simulink model "smartCart5_1work"  (R2016a)
settings: Solver=FixedStepDiscrete  StartTime=0.0  StopTime=inf  FixedStep=1  RelTol=1e-3
libraries: simulink x213, hdlsllib x84
(part 3 of 4)

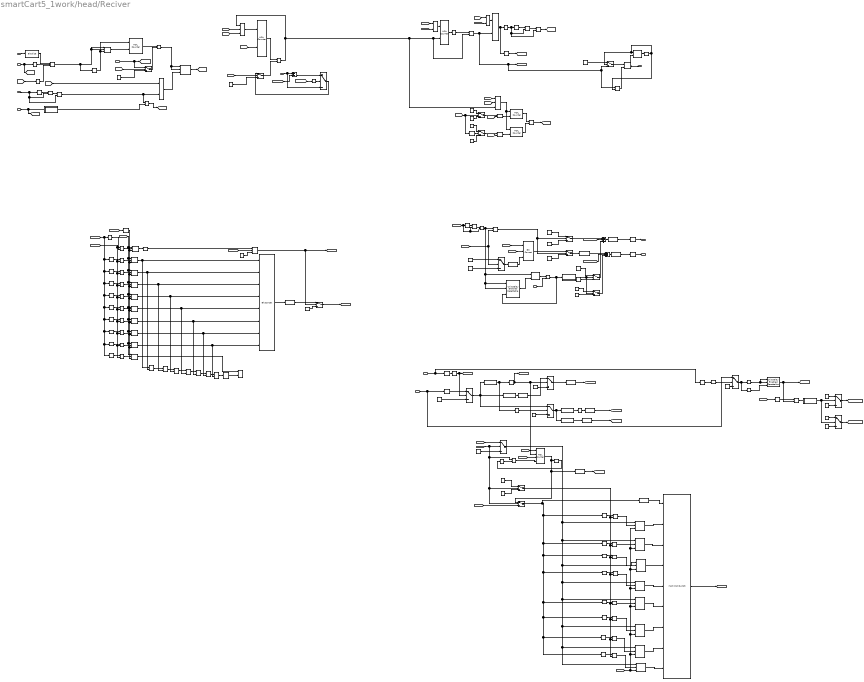
== system smartCart5_1work/head/Reciver ==
  note: Cхема формирования байта и проверка четности
  note: Схема связи (5)
  note: Схема формирования отчёта о работе приёмника (4)
  note: cхема управления и синхронизации (2)
  note: Схема обнаружение сообщения (1)
  RST : Inport  OutDataTypeStr=fixdt(1,3,0)
  IO : Inport  Port=2  OutDataTypeStr=boolean
  STOP : Inport  Port=3  OutDataTypeStr=boolean
  adr_IN : Inport  Port=4  OutDataTypeStr=uint8
  data_in : Inport  Port=5  OutDataTypeStr=uint32
  ON_RECIVER : Inport  Port=6  OutDataTypeStr=boolean
  TimOUT : Inport  Port=7  OutDataTypeStr=uint32
  time_transmite : Inport  Port=8  OutDataTypeStr=uint32
  time_transition : Inport  Port=9  OutDataTypeStr=uint32
  Add : Sum  Inputs=+++
  Add1 : Sum  Inputs=+++
  Add2 : Sum  Inputs=+-
  Bit Concat : hdlsllib/HDL Operations/Bit Concat  numInputs=8
  Bit Concat1 : hdlsllib/HDL Operations/Bit Concat  numInputs=3
  Bit Slice1 : hdlsllib/HDL Operations/Bit Slice  lidx=2  ridx=2
  Bit Slice2 : hdlsllib/HDL Operations/Bit Slice  lidx=1  ridx=0
  Bit Slice3 : hdlsllib/HDL Operations/Bit Slice  lidx=7  ridx=2
  Bit Slice4 : hdlsllib/HDL Operations/Bit Slice  lidx=2  ridx=2
  Bit Slice5 : hdlsllib/HDL Operations/Bit Slice  lidx=8  ridx=3
  Compare To Constant{1,3..4,13,21,31..33} (8 alike) : simulink/Logic and Bit Operations/Compare To Constant  relop===  const=0  OutDataTypeStr=boolean
  Compare To Constant10 : simulink/Logic and Bit Operations/Compare To Constant  relop===  const=7  OutDataTypeStr=boolean
  Compare To Constant11 : simulink/Logic and Bit Operations/Compare To Constant  relop===  const=8  OutDataTypeStr=boolean
  Compare To Constant12 : simulink/Logic and Bit Operations/Compare To Constant  relop===  const=9  OutDataTypeStr=boolean
  Compare To Constant14 : simulink/Logic and Bit Operations/Compare To Constant  relop===  const=6  OutDataTypeStr=boolean
  Compare To Constant15 : simulink/Logic and Bit Operations/Compare To Constant  relop===  const=7  OutDataTypeStr=boolean
  Compare To Constant{5,16,18,20,22,30} (6 alike) : simulink/Logic and Bit Operations/Compare To Constant  relop===  const=1  OutDataTypeStr=boolean
  Compare To Constant17 : simulink/Logic and Bit Operations/Compare To Constant  relop===  const=200  OutDataTypeStr=boolean
  Compare To Constant19 : simulink/Logic and Bit Operations/Compare To Constant  relop===  const=2  OutDataTypeStr=boolean
  Compare To Constant2 : simulink/Logic and Bit Operations/Compare To Constant  relop===  const=10  OutDataTypeStr=boolean
  Compare To Constant23 : simulink/Logic and Bit Operations/Compare To Constant  relop===  const=2  OutDataTypeStr=boolean
  Compare To Constant24 : simulink/Logic and Bit Operations/Compare To Constant  relop===  const=3  OutDataTypeStr=boolean
  Compare To Constant25 : simulink/Logic and Bit Operations/Compare To Constant  relop===  const=4  OutDataTypeStr=boolean
  Compare To Constant26 : simulink/Logic and Bit Operations/Compare To Constant  relop===  const=5  OutDataTypeStr=boolean
  Compare To Constant27 : simulink/Logic and Bit Operations/Compare To Constant  relop===  const=6  OutDataTypeStr=boolean
  Compare To Constant28 : simulink/Logic and Bit Operations/Compare To Constant  relop===  const=7  OutDataTypeStr=boolean
  Compare To Constant29 : simulink/Logic and Bit Operations/Compare To Constant  relop===  const=5  OutDataTypeStr=boolean
  Compare To Constant6 : simulink/Logic and Bit Operations/Compare To Constant  relop===  const=2  OutDataTypeStr=boolean
  Compare To Constant7 : simulink/Logic and Bit Operations/Compare To Constant  relop===  const=3  OutDataTypeStr=boolean
  Compare To Constant8 : simulink/Logic and Bit Operations/Compare To Constant  relop===  const=4  OutDataTypeStr=boolean
  Compare To Constant9 : simulink/Logic and Bit Operations/Compare To Constant  relop===  const=5  OutDataTypeStr=boolean
  Constant{,1,12,20} (4 alike) : Constant  Value=0  OutDataTypeStr=uint8
  Constant10 : Constant  Value=0  OutDataTypeStr=boolean  SampleTime=-1
  Constant11 : Constant  Value=0  OutDataTypeStr=boolean
  Constant{3,7,13..15} (5 alike) : Constant  Value=0  OutDataTypeStr=uint32  SampleTime=-1
  Constant16 : Constant  Value=0  OutDataTypeStr=uint8  SampleTime=-1
  Constant17 : Constant  Value=5  OutDataTypeStr=uint8  SampleTime=-1
  Constant18 : Constant  OutDataTypeStr=uint8  SampleTime=-1
  Constant19 : Constant  Value=6  OutDataTypeStr=uint8
  Constant2 : Constant  OutDataTypeStr=uint8
  Constant21 : Constant  Value=0  OutDataTypeStr=uint32
  Constant22 : Constant  OutDataTypeStr=uint32
  Constant23 : Constant  OutDataTypeStr=uint32  SampleTime=-1
  Constant24 : Constant  OutDataTypeStr=uint32  SampleTime=-1
  Constant26 : Constant  OutDataTypeStr=boolean  SampleTime=-1
  Constant27 : Constant  OutDataTypeStr=boolean  SampleTime=-1
  Constant28 : Constant  Value=0  OutDataTypeStr=boolean  SampleTime=-1
  Constant29 : Constant  Value=0  OutDataTypeStr=boolean  SampleTime=-1
  Constant4 : Constant  Value=2  OutDataTypeStr=fixdt(0,2,0)
  Constant5 : Constant  Value=0  OutDataTypeStr=uint8  SampleTime=-1
  Constant6 : Constant  OutDataTypeStr=boolean
  Constant8 : Constant  OutDataTypeStr=fixdt(0,2,0)
  Constant9 : Constant  OutDataTypeStr=boolean
  Data Type Conversion : DataTypeConversion  OutDataTypeStr=uint8
  Data Type Conversion1 : DataTypeConversion  OutDataTypeStr=fixdt(0,5,0)
  Data Type Conversion10 : DataTypeConversion  OutDataTypeStr=uint8
  Data Type Conversion2 : DataTypeConversion  OutDataTypeStr=uint8
  Data Type Conversion3 : DataTypeConversion  OutDataTypeStr=boolean
  Data Type Conversion4 : DataTypeConversion  OutDataTypeStr=uint32
  Data Type Conversion5 : DataTypeConversion  OutDataTypeStr=uint32
  Data Type Conversion6 : DataTypeConversion  OutDataTypeStr=fixdt(0,5,0)
  Data Type Conversion7 : DataTypeConversion  OutDataTypeStr=fixdt(0,2,0)
  Data Type Conversion8 : DataTypeConversion  OutDataTypeStr=fixdt(1,4,0)
  Data Type Conversion9 : DataTypeConversion  OutDataTypeStr=uint32
  Delay{1..9,11} (10 alike) : Delay  DelayLength=1  InitialCondition=0
  HDL Counter{,6,8..9} (4 alike) : hdlsllib/HDL Operations/HDL Counter  CountType=Free running  CountInit=0  CountStep=1  CountMax=1  CountFromType=Initial value  CountFrom=0  CountResetPort=on  CountLoadPort=off  CountEnbPort=on  CountDirPort=off  CountDataType=Unsigned  CountWordLen=32  CountFracLen=0  CountSampTime=1
  HDL Counter1 : hdlsllib/HDL Operations/HDL Counter  CountType=Free running  CountInit=0  CountStep=1  CountMax=1  CountFromType=Initial value  CountFrom=0  CountResetPort=on  CountLoadPort=off  CountEnbPort=on  CountDirPort=off  CountDataType=Unsigned  CountWordLen=1  CountFracLen=0  CountSampTime=1
  HDL Counter2 : hdlsllib/HDL Operations/HDL Counter  CountType=Count limited  CountInit=0  CountStep=1  CountMax=10  CountFromType=Initial value  CountFrom=0  CountResetPort=on  CountLoadPort=off  CountEnbPort=on  CountDirPort=off  CountDataType=Unsigned  CountWordLen=4  CountFracLen=0  CountSampTime=1
  HDL Counter3 : hdlsllib/HDL Operations/HDL Counter  CountType=Free running  CountInit=0  CountStep=1  CountMax=1  CountFromType=Initial value  CountFrom=0  CountResetPort=on  CountLoadPort=on  CountEnbPort=on  CountDirPort=off  CountDataType=Unsigned  CountWordLen=5  CountFracLen=0  CountSampTime=1
  HDL Counter4 : hdlsllib/HDL Operations/HDL Counter  CountType=Free running  CountInit=0  CountStep=1  CountMax=1  CountFromType=Initial value  CountFrom=0  CountResetPort=on  CountLoadPort=off  CountEnbPort=on  CountDirPort=off  CountDataType=Unsigned  CountWordLen=8  CountFracLen=0  CountSampTime=1
  HDL Counter5 : hdlsllib/HDL Operations/HDL Counter  CountType=Free running  CountInit=0  CountStep=1  CountMax=25  CountFromType=Initial value  CountFrom=0  CountResetPort=on  CountLoadPort=off  CountEnbPort=on  CountDirPort=off  CountDataType=Unsigned  CountWordLen=32  CountFracLen=0  CountSampTime=1
  Index Vector : MultiPortSwitch  DataPortOrder=Zero-based contiguous  Inputs=8  zeroidx=on
  Logical Operator{,7,9,12..21,33,36,38..46,49..50} (26 alike) : Logic  AllPortsSameDT=off  OutDataTypeStr=boolean
  Logical Operator{1,10..11,34..35,48} (6 alike) : Logic  Operator=OR  AllPortsSameDT=off  OutDataTypeStr=boolean
  Logical Operator2 : Logic  Operator=NOT  Inputs=3  AllPortsSameDT=off  OutDataTypeStr=boolean
  Logical Operator22 : Logic  Inputs=3  AllPortsSameDT=off  OutDataTypeStr=boolean
  Logical Operator{5..6,23..24,26..30,32} (10 alike) : Logic  Operator=XOR  AllPortsSameDT=off  OutDataTypeStr=boolean
  Logical Operator25 : Logic  Inputs=3  AllPortsSameDT=off  OutDataTypeStr=boolean
  Logical Operator31 : Logic  Operator=NOT  AllPortsSameDT=off  OutDataTypeStr=boolean
  Logical Operator37 : Logic  Operator=NOT  AllPortsSameDT=off  OutDataTypeStr=boolean
  Logical Operator4 : Logic  Operator=NOT  Inputs=3  AllPortsSameDT=off  OutDataTypeStr=boolean
  Logical Operator47 : Logic  Operator=NOT  Inputs=3  AllPortsSameDT=off  OutDataTypeStr=boolean
  Logical Operator51 : Logic  Operator=OR  Inputs=3  AllPortsSameDT=off  OutDataTypeStr=boolean
  Logical Operator8 : Logic  Operator=OR  Inputs=3  AllPortsSameDT=off  OutDataTypeStr=boolean
  Relational Operator{,1..3} (4 alike) : RelationalOperator  Operator===  OutDataTypeStr=boolean
  Relational Operator5 : RelationalOperator  Operator=>  OutDataTypeStr=boolean
  SA12 : simulink/Additional Math & Discrete/Additional Discrete/Unit Delay Enabled  vinit=0  tsamp=-1
  Switch{,1..18,20..21} (21 alike) : Switch  Criteria=u2 ~= 0
  Unit Delay Enabled Resettable{,1..21} (22 alike) : simulink/Additional Math & Discrete/Additional Discrete/Unit Delay Enabled Resettable  vinit=0.0  tsamp=-1
  signal_edg : Subsystem  TreatAsAtomicUnit=on
  signal_edg5 : Subsystem  TreatAsAtomicUnit=on
  signal_edg6 : Subsystem  TreatAsAtomicUnit=on
  AddrOUT : Outport  OutDataTypeStr=uint8
  STATUS : Outport  Port=2  OutDataTypeStr=uint32
  Strob : Outport  Port=3  OutDataTypeStr=boolean
  wires:
  RST/1 -> Bit Slice1/1
  Bit Slice1/1 -> Logical Operator25/1
  [bait_done] -> Logical Operator1/1
  Logical Operator1/1 -> Unit Delay Enabled Resettable/3
  Unit Delay Enabled Resettable/1 -> [Mes_res]
  HDL Counter/1 -> Relational Operator2/1
  Relational Operator2/1 -> Logical Operator8/1, Logical Operator51/3, HDL Counter1/2, Logical Operator/2
  HDL Counter1/1 -> Compare To Constant1/1
  Compare To Constant1/1 -> Logical Operator/1
  HDL Counter2/1 -> Delay3/1, Compare To Constant2/1
  Compare To Constant2/1 -> Logical Operator7/2, Logical Operator6/2, Delay2/1
  Delay2/1 -> Logical Operator6/1
  Logical Operator6/1 -> Logical Operator7/1
  Logical Operator8/1 -> HDL Counter/1
  Logical Operator7/1 -> [bait_done]
  [bait_done] -> Logical Operator8/2
  [Mes_res] -> HDL Counter/2
  Delay1/1 -> Logical Operator5/1
  Logical Operator5/1 -> Logical Operator9/1
  STOP/1 -> Logical Operator9/2, Logical Operator5/2, Delay1/1
  Logical Operator9/1 -> Logical Operator48/1, Logical Operator1/2
  [RST] -> Logical Operator8/3
  Logical Operator10/1 -> HDL Counter1/1
  [bait_done] -> Logical Operator10/1
  [RST] -> Logical Operator10/2
  Logical Operator11/1 -> HDL Counter2/1
  [bait_done] -> Logical Operator11/1
  [RST] -> Logical Operator11/2
  Delay3/1 -> [Number_bit]
  Compare To Constant5/1 -> Logical Operator13/1
  Compare To Constant6/1 -> Logical Operator14/1
  Logical Operator14/1 -> Unit Delay Enabled Resettable3/2
  Compare To Constant7/1 -> Logical Operator15/1
  Compare To Constant8/1 -> Logical Operator16/1
  Compare To Constant9/1 -> Logical Operator17/1
  Logical Operator17/1 -> Unit Delay Enabled Resettable6/2
  Compare To Constant14/1 -> Logical Operator18/1
  Logical Operator18/1 -> Unit Delay Enabled Resettable7/2
  Compare To Constant10/1 -> Logical Operator19/1
  Compare To Constant11/1 -> Logical Operator20/1
  Compare To Constant12/1 -> Logical Operator21/1
  [Number_bit] -> Compare To Constant12/1, Compare To Constant11/1, Compare To Constant10/1, Compare To Constant14/1, Compare To Constant9/1, Compare To Constant8/1, Compare To Constant7/1, Compare To Constant6/1, Compare To Constant5/1, Compare To Constant3/1
  Unit Delay Enabled Resettable1/1 -> Compare To Constant13/1
  Compare To Constant13/1 -> Logical Operator22/1
  Compare To Constant3/1 -> Logical Operator12/2
  [Get_val] -> Logical Operator17/2, Logical Operator21/2, Logical Operator20/2, Logical Operator19/2, Logical Operator18/2, Logical Operator16/2, Logical Operator15/2, Logical Operator14/2, Logical Operator13/2, Logical Operator12/1
  [bait_done] -> Logical Operator22/2
  Unit Delay Enabled Resettable3/1 -> Logical Operator23/2, Bit Concat/2
  Unit Delay Enabled Resettable4/1 -> Logical Operator24/2, Bit Concat/3
  Unit Delay Enabled Resettable5/1 -> Logical Operator26/2, Bit Concat/4
  Unit Delay Enabled Resettable6/1 -> Logical Operator27/2, Bit Concat/5
  Unit Delay Enabled Resettable7/1 -> Logical Operator28/2, Bit Concat/6
  Unit Delay Enabled Resettable8/1 -> Logical Operator29/2, Bit Concat/7
  Unit Delay Enabled Resettable9/1 -> Logical Operator30/2, Bit Concat/8
  Unit Delay Enabled Resettable2/1 -> Logical Operator23/1, Bit Concat/1
  Logical Operator23/1 -> Logical Operator24/1
  Logical Operator24/1 -> Logical Operator26/1
  Logical Operator26/1 -> Logical Operator27/1
  Logical Operator27/1 -> Logical Operator28/1
  Logical Operator28/1 -> Logical Operator29/1
  Logical Operator29/1 -> Logical Operator30/1
  Logical Operator30/1 -> Logical Operator31/1
  Bit Concat/1 -> Data Type Conversion/1
  Logical Operator31/1 -> Relational Operator/2
  Unit Delay Enabled Resettable10/1 -> Relational Operator/1
  Logical Operator22/1 -> Switch1/2, [Error_bait]
  Data Type Conversion/1 -> Switch1/1
  Constant/1 -> Switch1/3
  Constant1/1 -> Switch2/3
  Constant2/1 -> Switch2/1
  Constant5/1 -> Switch4/3
  [Error_bait] -> Logical Operator36/1, Switch6/2, Switch5/2, Switch4/2
  [bait] -> Switch4/1
  HDL Counter3/1 -> Switch6/1, Data Type Conversion2/1, Compare To Constant15/1
  Logical Operator36/1 -> HDL Counter3/4
  Compare To Constant15/1 -> Logical Operator37/1
  Logical Operator37/1 -> Logical Operator36/2
  Data Type Conversion2/1 -> [Num_Count]
  Logical Operator35/1 -> Switch2/2, Switch3/2
  Delay5/1 -> Unit Delay Enabled Resettable10/3, Unit Delay Enabled Resettable9/3, Unit Delay Enabled Resettable8/3, Unit Delay Enabled Resettable7/3, Unit Delay Enabled Resettable6/3, Unit Delay Enabled Resettable5/3, Unit Delay Enabled Resettable4/3, Unit Delay Enabled Resettable3/3, Unit Delay Enabled Resettable2/3, Unit Delay Enabled Resettable1/3
  [bait_done] -> Delay5/1
  Logical Operator13/1 -> Unit Delay Enabled Resettable2/2
  Logical Operator12/1 -> Unit Delay Enabled Resettable1/2
  Logical Operator15/1 -> Unit Delay Enabled Resettable4/2
  Logical Operator16/1 -> Unit Delay Enabled Resettable5/2
  Logical Operator19/1 -> Unit Delay Enabled Resettable8/2
  Logical Operator21/1 -> Unit Delay Enabled Resettable10/2
  [data] -> Unit Delay Enabled Resettable10/1, Unit Delay Enabled Resettable9/1, Unit Delay Enabled Resettable8/1, Unit Delay Enabled Resettable7/1, Unit Delay Enabled Resettable6/1, Unit Delay Enabled Resettable5/1, Unit Delay Enabled Resettable4/1, Unit Delay Enabled Resettable3/1, Unit Delay Enabled Resettable2/1, Unit Delay Enabled Resettable1/1
  Logical Operator20/1 -> Unit Delay Enabled Resettable9/2
  Logical Operator/1 -> Logical Operator34/1, Switch8/3, [Get_val], HDL Counter2/2
  Switch8/1 -> SA12/1
  Constant10/1 -> Switch8/1
  SA12/1 -> Strob/1, HDL Counter4/2
  HDL Counter4/1 -> Compare To Constant17/1
  Compare To Constant17/1 -> Switch8/2, HDL Counter4/1, Logical Operator34/2
  Logical Operator34/1 -> SA12/2
  Constant11/1 -> Switch5/3
  Constant6/1 -> Switch5/1
  [addRd] -> Switch6/3
  Constant9/1 -> Logical Operator22/3
  Index Vector/1 -> [Read_Byte]
  Bit Concat1/1 -> Switch3/1
  Switch3/1 -> Data Type Conversion4/1
  [Num_Count] -> Bit Concat1/2
  Constant12/1 -> Switch3/3
  Bit Slice2/1 -> Compare To Constant19/1, Compare To Constant18/1
  Bit Slice3/1 -> Data Type Conversion5/1
  Data Type Conversion5/1 -> Switch7/1
  Constant3/1 -> Switch7/3
  Switch7/1 -> Data Type Conversion6/1
  Data Type Conversion6/1 -> [VAL_COUNT]
  Compare To Constant16/1 -> Switch11/2, [Send_com]
  Compare To Constant18/1 -> [WE], Switch7/2, HDL Counter3/2
  [VAL_COUNT] -> HDL Counter3/3
  Compare To Constant19/1 -> Switch9/2
  Constant7/1 -> Switch9/3
  Switch9/1 -> Bit Slice5/1, Bit Slice4/1
  Bit Slice4/1 -> Compare To Constant20/1
  Compare To Constant20/1 -> Data Type Conversion3/1
  Data Type Conversion3/1 -> [RD]
  Bit Slice5/1 -> Data Type Conversion1/1
  Data Type Conversion1/1 -> [addRd]
  Constant4/1 -> Switch10/1
  Constant8/1 -> Switch10/3
  Switch10/1 -> Data Type Conversion7/1
  Data Type Conversion7/1 -> Bit Concat1/3
  Delay7/1 -> Compare To Constant16/1
  adr_IN/1 -> Delay9/1, Delay7/1
  data_in/1 -> Switch12/1, Delay11/1
  Switch11/1 -> Bit Slice2/1, Switch9/1, Bit Slice3/1
  [Error_bait] -> Logical Operator32/2, Logical Operator33/2, Delay4/1
  Delay4/1 -> Logical Operator32/1
  Logical Operator32/1 -> Logical Operator33/1
  Logical Operator33/1 -> Unit Delay Enabled Resettable20/1, Unit Delay Enabled Resettable20/2, HDL Counter5/1, Logical Operator35/1
  Delay11/1 -> Switch11/1
  Constant14/1 -> Switch11/3
  [Read_Byte] -> Bit Concat1/1
  [RD] -> Switch10/2, Logical Operator35/2
  Compare To Constant21/1 -> Logical Operator39/1
  Logical Operator39/1 -> Unit Delay Enabled Resettable11/2
  Compare To Constant22/1 -> Logical Operator40/1
  Logical Operator40/1 -> Unit Delay Enabled Resettable12/2
  Compare To Constant23/1 -> Logical Operator41/1
  Logical Operator41/1 -> Unit Delay Enabled Resettable13/2
  Compare To Constant24/1 -> Logical Operator42/1
  Logical Operator42/1 -> Unit Delay Enabled Resettable14/2
  Compare To Constant25/1 -> Logical Operator43/1
  Logical Operator43/1 -> Unit Delay Enabled Resettable15/2
  Compare To Constant26/1 -> Logical Operator44/1
  Logical Operator44/1 -> Unit Delay Enabled Resettable16/2
  Compare To Constant27/1 -> Logical Operator45/1
  Logical Operator45/1 -> Unit Delay Enabled Resettable18/2
  Switch4/1 -> Unit Delay Enabled Resettable19/1, Unit Delay Enabled Resettable18/1, Unit Delay Enabled Resettable16/1, Unit Delay Enabled Resettable15/1, Unit Delay Enabled Resettable14/1, Unit Delay Enabled Resettable13/1, Unit Delay Enabled Resettable12/1, Unit Delay Enabled Resettable11/1
  Compare To Constant28/1 -> Logical Operator46/1
  Logical Operator46/1 -> Unit Delay Enabled Resettable19/2
  Unit Delay Enabled Resettable19/1 -> Index Vector/9
  Unit Delay Enabled Resettable18/1 -> Index Vector/8
  Unit Delay Enabled Resettable16/1 -> Index Vector/7
  Unit Delay Enabled Resettable15/1 -> Index Vector/6
  Unit Delay Enabled Resettable14/1 -> Index Vector/5
  Unit Delay Enabled Resettable13/1 -> Index Vector/4
  Unit Delay Enabled Resettable12/1 -> Index Vector/3
  Unit Delay Enabled Resettable11/1 -> Index Vector/2
  Data Type Conversion8/1 -> Index Vector/1
  Switch6/1 -> Data Type Conversion8/1, Compare To Constant28/1, Compare To Constant27/1, Compare To Constant26/1, Compare To Constant25/1, Compare To Constant24/1, Compare To Constant23/1, Compare To Constant22/1, Compare To Constant21/1
  Switch5/1 -> Logical Operator46/2, Logical Operator45/2, Logical Operator44/2, Logical Operator43/2, Logical Operator42/2, Logical Operator41/2, Logical Operator40/2, Logical Operator39/2
  [RST] -> Unit Delay Enabled Resettable13/3, Unit Delay Enabled Resettable11/3, Unit Delay Enabled Resettable12/3, Unit Delay Enabled Resettable14/3, Unit Delay Enabled Resettable15/3, Unit Delay Enabled Resettable16/3, Unit Delay Enabled Resettable18/3, Unit Delay Enabled Resettable19/3
  Delay9/1 -> Compare To Constant29/1
  Compare To Constant29/1 -> Switch12/2
  Constant13/1 -> Switch12/3
  Switch12/1 -> Compare To Constant32/1, Compare To Constant30/1
  Compare To Constant30/1 -> Unit Delay Enabled Resettable17/1, Unit Delay Enabled Resettable17/2
  signal_edg/1(Out1) -> Switch14/2, Switch13/2
  Constant15/1 -> Switch14/3
  Constant16/1 -> Switch13/3
  Constant17/1 -> Switch13/1
  Constant18/1 -> Switch14/1
  Compare To Constant32/1 -> Unit Delay Enabled Resettable17/3
  Unit Delay Enabled Resettable17/1 -> Logical Operator38/2, [detect_error]
  [data] -> Compare To Constant31/1
  Compare To Constant31/1 -> Logical Operator38/1
  Logical Operator38/1 -> signal_edg/1(In1)
  [detect_error] -> Logical Operator47/1
  Logical Operator47/1 -> Logical Operator25/3
  Switch13/1 -> [addr_detect_error]
  Switch14/1 -> [data_detect_error]
  Data Type Conversion4/1 -> Add/1
  Switch2/1 -> Add1/1
  [addr_detect_error] -> Add1/2
  [data_detect_error] -> Add/2
  Add/1 -> Data Type Conversion9/1
  Add1/1 -> Data Type Conversion10/1
  Switch1/1 -> [bait]
  ON_RECIVER/1 -> [on_reciver], signal_edg5/1(In1)
  signal_edg5/1(Out1) -> Logical Operator48/2
  Logical Operator48/1 -> [RST]
  [RST] -> HDL Counter3/1
  Unit Delay Enabled Resettable20/1 -> HDL Counter5/2
  HDL Counter5/1 -> Relational Operator1/1
  Relational Operator1/1 -> Unit Delay Enabled Resettable20/3, signal_edg6/1(In1)
  signal_edg6/1(Out1) -> Switch16/2, Switch15/2
  Constant19/1 -> Switch15/1
  Constant20/1 -> Switch15/3
  Constant21/1 -> Switch16/3
  Constant22/1 -> Switch16/1
  Data Type Conversion9/1 -> Delay6/1
  Data Type Conversion10/1 -> Delay8/1
  Delay8/1 -> AddrOUT/1
  Delay6/1 -> STATUS/1
  Switch15/1 -> Add1/3
  Switch16/1 -> Add/3
  TimOUT/1 -> Relational Operator1/2
  Constant23/1 -> Switch/3
  [on_reciver] -> Switch/2
  Switch/1 -> Relational Operator2/2
  Unit Delay Enabled Resettable21/1 -> HDL Counter6/2
  HDL Counter6/1 -> Relational Operator3/1
  Constant24/1 -> Switch17/3
  [on_reciver] -> Switch17/2
  time_transition/1 -> Switch17/1, [time_transition]
  Switch17/1 -> Relational Operator3/2
  Relational Operator3/1 -> Unit Delay Enabled Resettable/1, Unit Delay Enabled Resettable/2
  IO/1 -> [IO], Compare To Constant33/1
  Add2/1 -> Switch18/1
  [time_transition] -> Add2/2
  Compare To Constant4/1 -> Switch18/2
  [Number_bit] -> Compare To Constant4/1
  Logical Operator25/1 -> Logical Operator2/1, Unit Delay Enabled Resettable21/2, Unit Delay Enabled Resettable21/1
  Logical Operator2/1 -> Unit Delay Enabled Resettable21/3, HDL Counter6/1
  Compare To Constant33/1 -> Logical Operator25/2
  time_transmite/1 -> Switch18/3, Add2/1
  Switch18/1 -> Switch/1
  [IO] -> Logical Operator4/1, Switch20/2
  Logical Operator4/1 -> Switch21/2
  Constant26/1 -> Switch20/1
  Constant27/1 -> Switch21/1
  Constant28/1 -> Switch20/3
  Constant29/1 -> Switch21/3
  Switch20/1 -> Logical Operator49/1
  Logical Operator49/1 -> HDL Counter8/2
  [Mes_res] -> Logical Operator49/2
  Switch21/1 -> Logical Operator50/1
  Logical Operator50/1 -> HDL Counter9/2
  [Mes_res] -> Logical Operator50/2
  [RST] -> Logical Operator51/2
  [bait_done] -> Logical Operator51/1
  Logical Operator51/1 -> HDL Counter9/1, HDL Counter8/1
  HDL Counter8/1 -> Relational Operator5/1
  HDL Counter9/1 -> Relational Operator5/2
  Relational Operator5/1 -> [data]

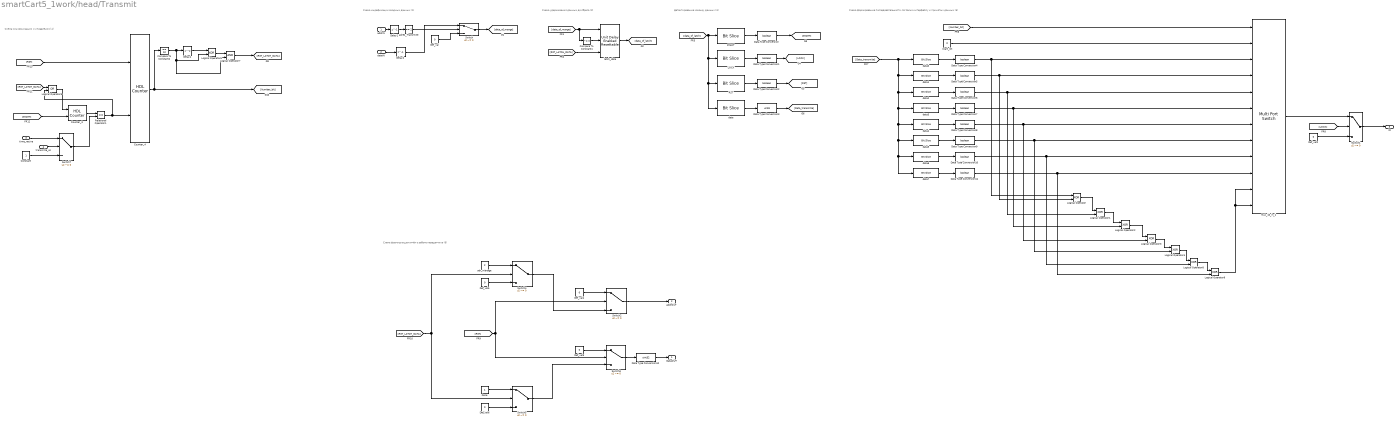
== system smartCart5_1work/head/Transmit ==
  note: Схема формирующая отчёт о работе передатчика (6)
  note: Схема формирование последовательности согласно интерфейсу и принятых данных (5)
  note: Детектирование команд, данных (3)
  note: Схема удерживания данных до сброса (2)
  note: Схема индефикации входных данных (1)
  note: Схема синхронизации и управления (4)
  addrIN : Inport  OutDataTypeStr=uint8
  dataIN : Inport  Port=2  OutDataTypeStr=fixdt(0,32,0)
  time_recive : Inport  Port=3  OutDataTypeStr=uint32
  transmite_on : Inport  Port=4  OutDataTypeStr=boolean
  Compare To Constant1 : simulink/Logic and Bit Operations/Compare To Constant  relop=~=  const=0  OutDataTypeStr=boolean
  Compare To Constant2 : simulink/Logic and Bit Operations/Compare To Constant  relop===  const=10  OutDataTypeStr=boolean
  Constant : Constant  OutDataTypeStr=uint32  SampleTime=-1
  Counter_3 : hdlsllib/HDL Operations/HDL Counter  CountType=Free running  CountInit=0  CountStep=1  CountMax=5208  CountFromType=Initial value  CountFrom=0  CountResetPort=on  CountLoadPort=off  CountEnbPort=on  CountDirPort=off  CountDataType=Unsigned  CountWordLen=32  CountFracLen=0  CountSampTime=1
  Counter_4 : hdlsllib/HDL Operations/HDL Counter  CountType=Count limited  CountInit=0  CountStep=1  CountMax=11  CountFromType=Initial value  CountFrom=0  CountResetPort=on  CountLoadPort=off  CountEnbPort=on  CountDirPort=off  CountDataType=Unsigned  CountWordLen=4  CountFracLen=0  CountSampTime=1
  Data Type Conversion{,1..2,4..11} (11 alike) : DataTypeConversion  OutDataTypeStr=boolean
  Data Type Conversion12 : DataTypeConversion  OutDataTypeStr=uint32
  Data Type Conversion3 : DataTypeConversion  OutDataTypeStr=uint8
  Def_val : Constant  Value=0  OutDataTypeStr=fixdt(0,32,0)  SampleTime=-1
  Def_val2 : Constant  Value=0  OutDataTypeStr=boolean  SampleTime=-1
  Def_val{3..6} (4 alike) : Constant  Value=0  OutDataTypeStr=uint8  SampleTime=-1
  Delay1 : Delay  DelayLength=1  InitialCondition=0
  Delay2 : Delay  DelayLength=1  InitialCondition=0
  Delay4 : Delay
  Done : Constant  OutDataTypeStr=uint8  SampleTime=-1
  LOCK : hdlsllib/HDL Operations/Bit Slice  lidx=1  ridx=1
  Logical Operator{,1..4,6,8..9} (8 alike) : Logic  Operator=XOR  AllPortsSameDT=off  OutDataTypeStr=boolean
  Logical Operator5 : Logic  Operator=OR  AllPortsSameDT=off  OutDataTypeStr=boolean
  Logical Operator7 : Logic  AllPortsSameDT=off  OutDataTypeStr=boolean
  RST : hdlsllib/HDL Operations/Bit Slice  lidx=2  ridx=2
  Relational Operator1 : RelationalOperator  Operator===  OutDataTypeStr=boolean
  START : hdlsllib/HDL Operations/Bit Slice  lidx=0  ridx=0
  Switch{,1..5,7} (7 alike) : Switch  Criteria=u2 ~= 0
  adr_manage : Constant  Value=2  OutDataTypeStr=uint8  SampleTime=-1
  adres_Transmite : simulink/Logic and Bit Operations/Compare To Constant  relop===  const=2  OutDataTypeStr=boolean
  data : hdlsllib/HDL Operations/Bit Slice  lidx=10  ridx=3
  "data0 " : hdlsllib/HDL Operations/Bit Slice  lidx=0  ridx=0
  data1 : hdlsllib/HDL Operations/Bit Slice  lidx=1  ridx=1
  data2 : hdlsllib/HDL Operations/Bit Slice  lidx=2  ridx=2
  data3 : hdlsllib/HDL Operations/Bit Slice  lidx=3  ridx=3
  data4 : hdlsllib/HDL Operations/Bit Slice  lidx=4  ridx=4
  data5 : hdlsllib/HDL Operations/Bit Slice  lidx=5  ridx=5
  data6 : hdlsllib/HDL Operations/Bit Slice  lidx=6  ridx=6
  data7 : hdlsllib/HDL Operations/Bit Slice  lidx=7  ridx=7
  latch_data : simulink/Additional Math & Discrete/Additional Discrete/Unit Delay Enabled Resettable  vinit=0  tsamp=-1
  mux_10_in_1 : MultiPortSwitch  DataPortOrder=Zero-based contiguous  Inputs=11  zeroidx=on
  start_bit : Constant  Value=0  OutDataTypeStr=boolean  SampleTime=-1
  DataOUT : Outport  OutDataTypeStr=uint32
  addrOUT : Outport  Port=2  OutDataTypeStr=uint8
  IO : Outport  Port=3  OutDataTypeStr=boolean
  wires:
  adres_Transmite/1 -> Switch/2
  Def_val/1 -> Switch/3
  START/1 -> Data Type Conversion/1
  LOCK/1 -> Data Type Conversion1/1
  RST/1 -> Data Type Conversion2/1
  data/1 -> Data Type Conversion3/1
  [RST_LATCH_DATA] -> latch_data/3
  Switch/1 -> [data_of_mange]
  latch_data/1 -> [data_of_latch]
  [data_of_latch] -> data/1, RST/1, LOCK/1, START/1
  Data Type Conversion/1 -> [START]
  Data Type Conversion1/1 -> [LOCK]
  Data Type Conversion2/1 -> [RST]
  Compare To Constant1/1 -> latch_data/2
  [Number_bit] -> mux_10_in_1/1
  start_bit/1 -> mux_10_in_1/2
  "data0 "/1 -> Data Type Conversion4/1
  data1/1 -> Data Type Conversion5/1
  data2/1 -> Data Type Conversion6/1
  data3/1 -> Data Type Conversion7/1
  data4/1 -> Data Type Conversion8/1
  data5/1 -> Data Type Conversion9/1
  data6/1 -> Data Type Conversion10/1
  [Data_transmite] -> data7/1, data6/1, data5/1, data4/1, data3/1, data2/1, data1/1, "data0 "/1
  data7/1 -> Data Type Conversion11/1
  mux_10_in_1/1 -> Switch1/1
  [LOCK] -> Switch1/2
  Switch1/1 -> IO/1
  Switch2/1 -> addrOUT/1
  Def_val4/1 -> Switch2/1
  Def_val3/1 -> Switch3/1
  [RST] -> Switch2/2, Switch3/2
  Switch4/1 -> Switch2/3
  Switch5/1 -> Switch3/3
  [RST_LATCH_DATA] -> Switch4/2, Switch5/2
  Def_val5/1 -> Switch4/3
  Def_val6/1 -> Switch5/3
  adr_manage/1 -> Switch4/1
  Done/1 -> Switch5/1
  [data_of_mange] -> latch_data/1, Compare To Constant1/1
  Data Type Conversion3/1 -> [Data_transmite]
  Def_val2/1 -> Switch1/3
  addrIN/1 -> Delay1/1
  Delay1/1 -> adres_Transmite/1
  dataIN/1 -> Delay2/1
  Delay2/1 -> Switch/1
  Data Type Conversion12/1 -> DataOUT/1
  Switch3/1 -> Data Type Conversion12/1
  Counter_3/1 -> Relational Operator1/1
  Relational Operator1/1 -> Logical Operator5/2, Counter_4/2
  Counter_4/1 -> Compare To Constant2/1, [Number_bit]
  [START] -> Counter_3/2
  Compare To Constant2/1 -> Logical Operator7/2, Logical Operator6/2, Delay4/1
  Delay4/1 -> Logical Operator6/1
  Logical Operator6/1 -> Logical Operator7/1
  Logical Operator7/1 -> [RST_LATCH_DATA]
  Constant/1 -> Switch7/3
  Switch7/1 -> Relational Operator1/2
  [RST] -> Counter_4/1
  time_recive/1 -> Switch7/1
  transmite_on/1 -> Switch7/2
  [RST_LATCH_DATA] -> Logical Operator5/1
  Logical Operator5/1 -> Counter_3/1
  Logical Operator/1 -> Logical Operator1/1
  Logical Operator1/1 -> Logical Operator2/1
  Logical Operator2/1 -> Logical Operator3/1
  Logical Operator3/1 -> Logical Operator4/1
  Logical Operator4/1 -> Logical Operator8/1
  Logical Operator8/1 -> Logical Operator9/1
  Data Type Conversion4/1 -> Logical Operator/1, mux_10_in_1/3
  Data Type Conversion5/1 -> Logical Operator/2, mux_10_in_1/4
  Data Type Conversion6/1 -> Logical Operator1/2, mux_10_in_1/5
  Data Type Conversion7/1 -> Logical Operator2/2, mux_10_in_1/6
  Data Type Conversion8/1 -> mux_10_in_1/7, Logical Operator3/2
  Data Type Conversion9/1 -> Logical Operator4/2, mux_10_in_1/8
  Data Type Conversion10/1 -> Logical Operator8/2, mux_10_in_1/9
  Data Type Conversion11/1 -> Logical Operator9/2, mux_10_in_1/10
  Logical Operator9/1 -> mux_10_in_1/11, mux_10_in_1/12

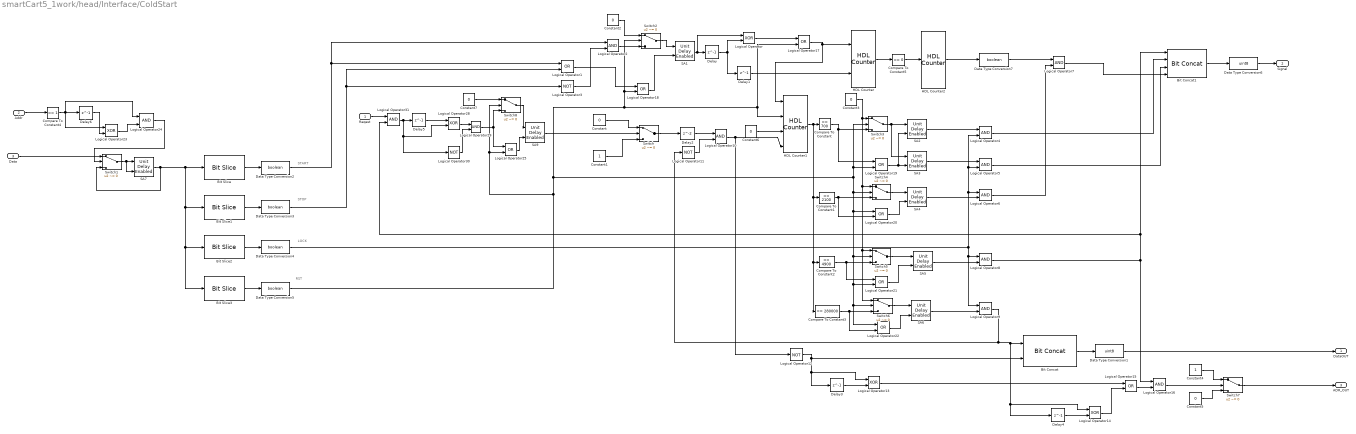
== system smartCart5_1work/head/Interface/ColdStart ==
  note: RST
  note: START
  note: STOP
  note: LOCK
  Reqest : Inport  OutDataTypeStr=boolean
  Addr : Inport  Port=2  OutDataTypeStr=uint8
  Data : Inport  Port=3  OutDataTypeStr=uint8
  Bit Concat : hdlsllib/HDL Operations/Bit Concat  numInputs=2
  Bit Concat1 : hdlsllib/HDL Operations/Bit Concat  numInputs=4
  Bit Slice : hdlsllib/HDL Operations/Bit Slice  lidx=3  ridx=3
  Bit Slice1 : hdlsllib/HDL Operations/Bit Slice  lidx=2  ridx=2
  Bit Slice2 : hdlsllib/HDL Operations/Bit Slice  lidx=1  ridx=1
  Bit Slice3 : hdlsllib/HDL Operations/Bit Slice  lidx=0  ridx=0
  Compare To Constant : simulink/Logic and Bit Operations/Compare To Constant  relop===  const=700  OutDataTypeStr=boolean
  Compare To Constant1 : simulink/Logic and Bit Operations/Compare To Constant  relop===  const=2100  OutDataTypeStr=boolean
  Compare To Constant2 : simulink/Logic and Bit Operations/Compare To Constant  relop===  const=4900  OutDataTypeStr=boolean
  Compare To Constant3 : simulink/Logic and Bit Operations/Compare To Constant  relop===  const=280000  OutDataTypeStr=boolean
  Compare To Constant4 : simulink/Logic and Bit Operations/Compare To Constant  relop===  const=1  OutDataTypeStr=boolean
  Compare To Constant5 : simulink/Logic and Bit Operations/Compare To Constant  relop===  const=0  OutDataTypeStr=boolean
  Constant{,2..3,7} (4 alike) : Constant  Value=0  OutDataTypeStr=boolean
  Constant1 : Constant  OutDataTypeStr=boolean
  Constant4 : Constant  OutDataTypeStr=uint8
  Constant5 : Constant  Value=0  OutDataTypeStr=uint8
  Constant6 : Constant  Value=0  OutDataTypeStr=fixdt(0,32,0)
  Data Type Conversion1 : DataTypeConversion  OutDataTypeStr=uint8
  Data Type Conversion{2..5,7} (5 alike) : DataTypeConversion  OutDataTypeStr=boolean
  Data Type Conversion6 : DataTypeConversion  OutDataTypeStr=uint8
  Delay{,1,3..6} (6 alike) : Delay  DelayLength=1  InitialCondition=0
  Delay2 : Delay  InitialCondition=0
  HDL Counter : hdlsllib/HDL Operations/HDL Counter  CountType=Count limited  CountInit=0  CountStep=1  CountMax=6  CountFromType=Initial value  CountFrom=0  CountResetPort=on  CountLoadPort=off  CountEnbPort=on  CountDirPort=off  CountDataType=Unsigned  CountWordLen=3  CountFracLen=0  CountSampTime=277e-9
  HDL Counter1 : hdlsllib/HDL Operations/HDL Counter  CountType=Count limited  CountInit=0  CountStep=1  CountMax=40000  CountFromType=Initial value  CountFrom=0  CountResetPort=on  CountLoadPort=on  CountEnbPort=on  CountDirPort=off  CountDataType=Unsigned  CountWordLen=32  CountFracLen=0  CountSampTime=277e-9
  HDL Counter2 : hdlsllib/HDL Operations/HDL Counter  CountType=Free running  CountInit=0  CountStep=1  CountMax=5  CountFromType=Initial value  CountFrom=0  CountResetPort=off  CountLoadPort=off  CountEnbPort=on  CountDirPort=off  CountDataType=Unsigned  CountWordLen=1  CountFracLen=0  CountSampTime=277e-9
  Logical Operator{,13..14,23,28} (5 alike) : Logic  Operator=XOR  AllPortsSameDT=off  OutDataTypeStr=boolean
  Logical Operator{1,15,17..22,25} (9 alike) : Logic  Operator=OR  AllPortsSameDT=off  OutDataTypeStr=boolean
  Logical Operator{2,4..10,16,24,29,31} (12 alike) : Logic  AllPortsSameDT=off  OutDataTypeStr=boolean
  Logical Operator{3,11..12,30} (4 alike) : Logic  Operator=NOT  AllPortsSameDT=off  OutDataTypeStr=boolean
  SA{1..7,9} (8 alike) : simulink/Additional Math & Discrete/Additional Discrete/Unit Delay Enabled  vinit=0  tsamp=-1
  Switch{,1..8} (9 alike) : Switch  Criteria=u2 ~= 0
  DataOUT : Outport  OutDataTypeStr=uint8
  Signal : Outport  Port=2  OutDataTypeStr=uint8
  ADR_OUT : Outport  Port=3  OutDataTypeStr=uint8
  wires:
  SA1/1 -> Logical Operator/1, Delay/1
  Delay/1 -> Delay1/1, Logical Operator/2
  Constant/1 -> Switch/1
  Constant1/1 -> Switch/3
  Logical Operator3/1 -> Logical Operator2/2
  Switch/1 -> Delay2/1
  SA2/1 -> Logical Operator4/1
  Logical Operator4/1 -> Bit Concat1/2
  SA3/1 -> Logical Operator5/1
  SA4/1 -> Logical Operator6/2
  Logical Operator6/1 -> Logical Operator7/2
  SA5/1 -> Logical Operator8/2
  Data Type Conversion2/1 -> Logical Operator2/1, Logical Operator1/1
  Data Type Conversion3/1 -> Logical Operator3/1, Logical Operator1/2
  Data Type Conversion4/1 -> Logical Operator8/1, Logical Operator9/1, Logical Operator4/2, Logical Operator5/2, Logical Operator6/1
  SA6/1 -> Logical Operator9/2
  Delay2/1 -> Logical Operator10/1
  Logical Operator11/1 -> Logical Operator10/2
  Bit Concat/1 -> Data Type Conversion1/1
  Logical Operator12/1 -> Logical Operator13/1, Delay3/1, Bit Concat/2
  Delay3/1 -> Logical Operator13/2
  Logical Operator9/1 -> Logical Operator11/1, Bit Concat/1, Logical Operator14/1, Delay4/1
  Delay4/1 -> Logical Operator14/2
  Logical Operator13/1 -> Logical Operator15/1
  Logical Operator14/1 -> Logical Operator15/2
  Logical Operator15/1 -> Logical Operator16/2
  Switch1/1 -> SA7/2, SA7/1
  SA7/1 -> Bit Slice/1, Bit Slice3/1, Bit Slice2/1, Bit Slice1/1, Switch1/3
  Bit Slice/1 -> Data Type Conversion2/1
  Bit Slice1/1 -> Data Type Conversion3/1
  Bit Slice2/1 -> Data Type Conversion4/1
  Bit Slice3/1 -> Data Type Conversion5/1
  Logical Operator/1 -> Logical Operator17/1
  Logical Operator17/1 -> HDL Counter1/1, HDL Counter/1
  Logical Operator1/1 -> Logical Operator18/1
  Logical Operator18/1 -> SA1/2
  Switch2/1 -> SA1/1
  Logical Operator2/1 -> Switch2/3
  Constant2/1 -> Switch2/1
  Switch3/1 -> SA3/1, SA2/1
  Switch4/1 -> SA4/1
  Switch5/1 -> SA5/1
  Switch6/1 -> SA6/1
  Constant3/1 -> Switch4/1, Switch6/1, Switch5/1, Switch3/1
  Logical Operator19/1 -> SA2/2, SA3/2
  Logical Operator20/1 -> SA4/2
  Compare To Constant/1 -> Switch3/3, Logical Operator19/1
  Compare To Constant1/1 -> Logical Operator20/2, Switch4/3
  Compare To Constant2/1 -> Logical Operator21/1, Switch5/3
  Logical Operator21/1 -> SA5/2
  Compare To Constant3/1 -> Logical Operator22/2, Switch6/3
  Logical Operator22/1 -> SA6/2
  Logical Operator7/1 -> Bit Concat1/4
  Bit Concat1/1 -> Data Type Conversion6/1
  Logical Operator16/1 -> Switch7/2
  Constant4/1 -> Switch7/1
  Constant5/1 -> Switch7/3
  Data/1 -> Switch1/1
  Addr/1 -> Compare To Constant4/1
  Data Type Conversion6/1 -> Signal/1
  Logical Operator10/1 -> HDL Counter1/4, Logical Operator12/1
  Delay1/1 -> HDL Counter/2
  HDL Counter2/1 -> Data Type Conversion7/1
  Data Type Conversion7/1 -> Logical Operator7/1
  Compare To Constant5/1 -> HDL Counter2/1
  HDL Counter/1 -> Compare To Constant5/1
  Delay5/1 -> Logical Operator28/1
  Logical Operator28/1 -> Logical Operator29/1
  Logical Operator30/1 -> Logical Operator29/2
  Logical Operator29/1 -> Switch8/3, Logical Operator25/1
  Reqest/1 -> Logical Operator31/1
  Logical Operator31/1 -> Logical Operator28/2, Logical Operator30/1, Delay5/1
  SA9/1 -> Switch/2
  Data Type Conversion1/1 -> DataOUT/1
  Data Type Conversion5/1 -> Logical Operator25/2, Switch8/2, Switch4/2, Logical Operator20/1, Logical Operator21/2, Logical Operator22/1, Switch6/2, Switch5/2, Logical Operator19/2, Switch3/2, Logical Operator17/2, HDL Counter1/2, Switch2/2, Logical Operator18/2
  Switch7/1 -> ADR_OUT/1
  Compare To Constant4/1 -> Logical Operator24/1, Logical Operator23/1, Delay6/1
  Delay6/1 -> Logical Operator23/2
  Logical Operator23/1 -> Logical Operator24/2
  Logical Operator24/1 -> Switch1/2
  Logical Operator8/1 -> Logical Operator31/2, Bit Concat1/1, Logical Operator16/1
  Constant6/1 -> HDL Counter1/3
  Logical Operator25/1 -> SA9/2
  Switch8/1 -> SA9/1
  Constant7/1 -> Switch8/1
  HDL Counter1/1 -> Compare To Constant3/1, Compare To Constant2/1, Compare To Constant1/1, Compare To Constant/1
  Logical Operator5/1 -> Bit Concat1/3

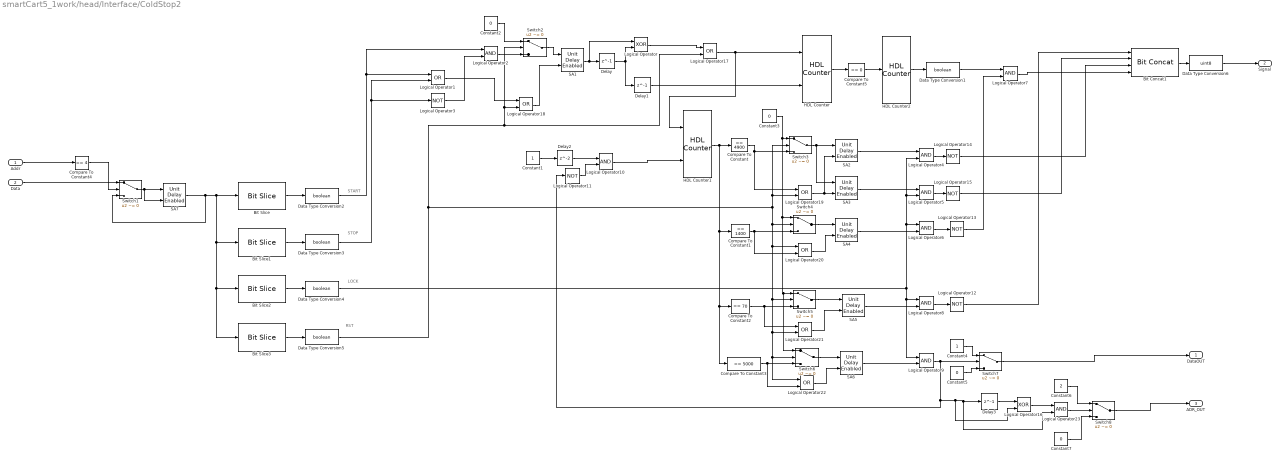
== system smartCart5_1work/head/Interface/ColdStop2 ==
  note: RST
  note: START
  note: STOP
  note: LOCK
  Addr : Inport  OutDataTypeStr=uint8
  Data : Inport  Port=2  OutDataTypeStr=uint8
  Bit Concat1 : hdlsllib/HDL Operations/Bit Concat  numInputs=4
  Bit Slice : hdlsllib/HDL Operations/Bit Slice  lidx=3  ridx=3
  Bit Slice1 : hdlsllib/HDL Operations/Bit Slice  lidx=2  ridx=2
  Bit Slice2 : hdlsllib/HDL Operations/Bit Slice  lidx=1  ridx=1
  Bit Slice3 : hdlsllib/HDL Operations/Bit Slice  lidx=0  ridx=0
  Compare To Constant : simulink/Logic and Bit Operations/Compare To Constant  relop===  const=4900  OutDataTypeStr=boolean
  Compare To Constant1 : simulink/Logic and Bit Operations/Compare To Constant  relop===  const=1400  OutDataTypeStr=boolean
  Compare To Constant2 : simulink/Logic and Bit Operations/Compare To Constant  relop===  const=70  OutDataTypeStr=boolean
  Compare To Constant3 : simulink/Logic and Bit Operations/Compare To Constant  relop===  const=5000  OutDataTypeStr=boolean
  Compare To Constant4 : simulink/Logic and Bit Operations/Compare To Constant  relop===  const=4  OutDataTypeStr=boolean
  Compare To Constant5 : simulink/Logic and Bit Operations/Compare To Constant  relop===  const=0  OutDataTypeStr=boolean
  Constant1 : Constant  OutDataTypeStr=boolean
  Constant2 : Constant  Value=0  OutDataTypeStr=boolean
  Constant3 : Constant  Value=0  OutDataTypeStr=boolean
  Constant4 : Constant  OutDataTypeStr=uint8
  Constant5 : Constant  Value=0  OutDataTypeStr=uint8
  Constant6 : Constant  Value=2  OutDataTypeStr=uint8
  Constant7 : Constant  Value=0  OutDataTypeStr=uint8
  Data Type Conversion{1..5} (5 alike) : DataTypeConversion  OutDataTypeStr=boolean
  Data Type Conversion6 : DataTypeConversion  OutDataTypeStr=uint8
  Delay : Delay  DelayLength=1  InitialCondition=0
  Delay1 : Delay  DelayLength=1  InitialCondition=0
  Delay2 : Delay  InitialCondition=0
  Delay3 : Delay  DelayLength=1  InitialCondition=0
  HDL Counter : hdlsllib/HDL Operations/HDL Counter  CountType=Count limited  CountInit=0  CountStep=1  CountMax=6  CountFromType=Initial value  CountFrom=0  CountResetPort=on  CountLoadPort=off  CountEnbPort=on  CountDirPort=off  CountDataType=Unsigned  CountWordLen=3  CountFracLen=0  CountSampTime=277e-9
  HDL Counter1 : hdlsllib/HDL Operations/HDL Counter  CountType=Count limited  CountInit=0  CountStep=1  CountMax=40000  CountFromType=Initial value  CountFrom=0  CountResetPort=on  CountLoadPort=off  CountEnbPort=on  CountDirPort=off  CountDataType=Unsigned  CountWordLen=32  CountFracLen=0  CountSampTime=277e-9
  HDL Counter2 : hdlsllib/HDL Operations/HDL Counter  CountType=Free running  CountInit=0  CountStep=1  CountMax=6  CountFromType=Initial value  CountFrom=0  CountResetPort=off  CountLoadPort=off  CountEnbPort=on  CountDirPort=off  CountDataType=Unsigned  CountWordLen=1  CountFracLen=0  CountSampTime=277e-9
  Logical Operator : Logic  Operator=XOR  AllPortsSameDT=off  OutDataTypeStr=boolean
  Logical Operator{1,17..22} (7 alike) : Logic  Operator=OR  AllPortsSameDT=off  OutDataTypeStr=boolean
  Logical Operator{2,4..10,23} (9 alike) : Logic  AllPortsSameDT=off  OutDataTypeStr=boolean
  Logical Operator{3,11..15} (6 alike) : Logic  Operator=NOT  AllPortsSameDT=off  OutDataTypeStr=boolean
  Logical Operator16 : Logic  Operator=XOR  AllPortsSameDT=off  OutDataTypeStr=boolean
  SA{1..7} (7 alike) : simulink/Additional Math & Discrete/Additional Discrete/Unit Delay Enabled  vinit=0  tsamp=-1
  Switch{1..8} (8 alike) : Switch  Criteria=u2 ~= 0
  DataOUT : Outport  OutDataTypeStr=uint8
  Signal : Outport  Port=2  OutDataTypeStr=uint8
  ADR_OUT : Outport  Port=3  OutDataTypeStr=uint8
  wires:
  SA1/1 -> Logical Operator/1, Delay/1
  Delay/1 -> Delay1/1, Logical Operator/2
  Logical Operator3/1 -> Logical Operator2/2
  Constant1/1 -> Delay2/1
  HDL Counter1/1 -> Compare To Constant3/1, Compare To Constant2/1, Compare To Constant1/1, Compare To Constant/1
  SA2/1 -> Logical Operator4/1
  SA3/1 -> Logical Operator5/1
  SA4/1 -> Logical Operator6/2
  SA5/1 -> Logical Operator8/2
  Data Type Conversion2/1 -> Logical Operator2/1, Logical Operator1/1
  Data Type Conversion3/1 -> Logical Operator3/1, Logical Operator1/2
  Data Type Conversion4/1 -> Logical Operator8/1, Logical Operator9/1, Logical Operator4/2, Logical Operator5/2, Logical Operator6/1
  SA6/1 -> Logical Operator9/2
  Delay2/1 -> Logical Operator10/1
  Logical Operator11/1 -> Logical Operator10/2
  Logical Operator9/1 -> Logical Operator11/1, Logical Operator16/2, Logical Operator23/2, Delay3/1, Switch7/2
  Compare To Constant4/1 -> Switch1/2
  Switch1/1 -> SA7/2, SA7/1
  SA7/1 -> Bit Slice3/1, Bit Slice2/1, Bit Slice1/1, Bit Slice/1, Switch1/3
  Bit Slice/1 -> Data Type Conversion2/1
  Bit Slice1/1 -> Data Type Conversion3/1
  Bit Slice2/1 -> Data Type Conversion4/1
  Bit Slice3/1 -> Data Type Conversion5/1
  Logical Operator/1 -> Logical Operator17/1
  Logical Operator17/1 -> HDL Counter1/1, HDL Counter/1
  Data Type Conversion5/1 -> Switch4/2, Logical Operator20/1, Logical Operator21/2, Logical Operator22/1, Switch6/2, Switch5/2, Logical Operator19/2, Switch3/2, Logical Operator17/2, Switch2/2, Logical Operator18/2
  Logical Operator1/1 -> Logical Operator18/1
  Logical Operator18/1 -> SA1/2
  Switch2/1 -> SA1/1
  Logical Operator2/1 -> Switch2/3
  Constant2/1 -> Switch2/1
  Switch3/1 -> SA3/1, SA2/1
  Switch4/1 -> SA4/1
  Switch5/1 -> SA5/1
  Switch6/1 -> SA6/1
  Constant3/1 -> Switch4/1, Switch6/1, Switch5/1, Switch3/1
  Logical Operator19/1 -> SA2/2, SA3/2
  Logical Operator20/1 -> SA4/2
  Compare To Constant/1 -> Switch3/3, Logical Operator19/1
  Compare To Constant1/1 -> Logical Operator20/2, Switch4/3
  Compare To Constant2/1 -> Logical Operator21/1, Switch5/3
  Logical Operator21/1 -> SA5/2
  Compare To Constant3/1 -> Logical Operator22/2, Switch6/3
  Logical Operator22/1 -> SA6/2
  Logical Operator7/1 -> Bit Concat1/4
  Bit Concat1/1 -> Data Type Conversion6/1
  Logical Operator8/1 -> Logical Operator12/1
  Logical Operator12/1 -> Bit Concat1/1
  Logical Operator6/1 -> Logical Operator13/1
  Logical Operator13/1 -> Logical Operator7/2
  Logical Operator4/1 -> Logical Operator14/1
  Logical Operator14/1 -> Bit Concat1/3
  Logical Operator5/1 -> Logical Operator15/1
  Logical Operator15/1 -> Bit Concat1/2
  Constant4/1 -> Switch7/1
  Constant5/1 -> Switch7/3
  Delay3/1 -> Logical Operator16/1
  Logical Operator16/1 -> Logical Operator23/1
  Logical Operator23/1 -> Switch8/2
  Constant6/1 -> Switch8/1
  Constant7/1 -> Switch8/3
  Data Type Conversion6/1 -> Signal/1
  Delay1/1 -> HDL Counter/2
  Logical Operator10/1 -> HDL Counter1/2
  Data Type Conversion1/1 -> Logical Operator7/1
  HDL Counter/1 -> Compare To Constant5/1
  Compare To Constant5/1 -> HDL Counter2/1
  HDL Counter2/1 -> Data Type Conversion1/1
  Data/1 -> Switch1/1
  Addr/1 -> Compare To Constant4/1
  Switch7/1 -> DataOUT/1
  Switch8/1 -> ADR_OUT/1
